simulink model "lyapanovPID"  (R2018b)
settings: Solver=VariableStepAuto  StartTime=0.0  StopTime=100  RelTol=1e-3
undefined symbols (not defined in the file or in its folder): DiscIntNeverNeededParam
libraries: simulink x1
settings Model: Creator=erfan  LastModifiedBy=erfan

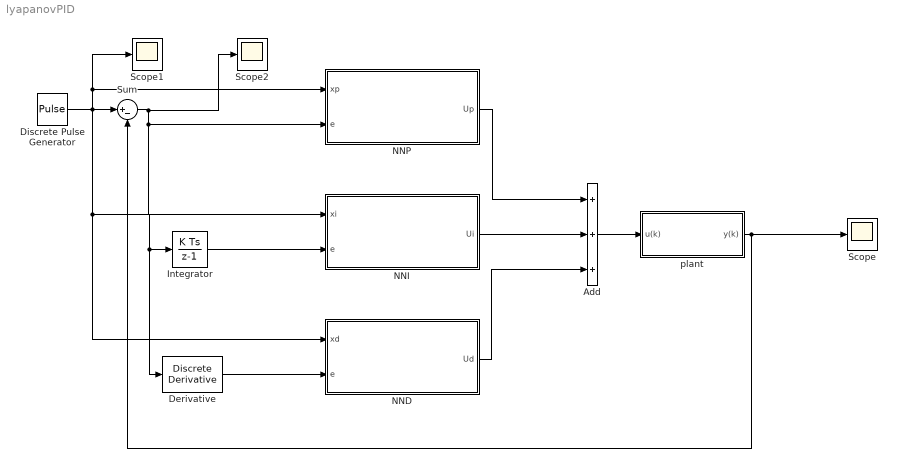
== system lyapanovPID ==
  Add : Sum  Inputs=+++
  Derivative : simulink/Quick Insert/Discrete/Discrete Derivative  gainval=1.0  ICPrevScaledInput=0.0  OutMin=[]  OutMax=[]  OutDataType=fixdt(1, 16)  OutScaling=2^-10  DoSatur=off
      settings: SourceProductName=Simulink  SourceProductBaseCode=SL
  Discrete Pulse Generator : DiscretePulseGenerator  Period=10  PulseWidth=5
  Integrator : DiscreteIntegrator  SampleTime=-1  ICPrevOutput=DiscIntNeverNeededParam  ICPrevScaledInput=DiscIntNeverNeededParam
  NND : Subsystem
  NNI : Subsystem
  NNP : Subsystem
  Scope : Scope
  Scope1 : Scope
  Scope2 : Scope
  Sum : Sum  Inputs=|+-
  plant : Subsystem
  wires:
  Derivative/1 -> NND/2(e)
  Integrator/1 -> NNI/2(e)
  NNP/1(Up) -> Add/1
  NNI/1(Ui) -> Add/2
  NND/1(Ud) -> Add/3
  Add/1 -> plant/1(u(k))
  plant/1(y(k)) -> Sum/2, Scope/1
  Sum/1 -> Scope2/1, NNP/2(e), Derivative/1, Integrator/1
  Discrete Pulse Generator/1 -> NNP/1(xp), Scope1/1, NND/1(xd), NNI/1(xi), Sum/1

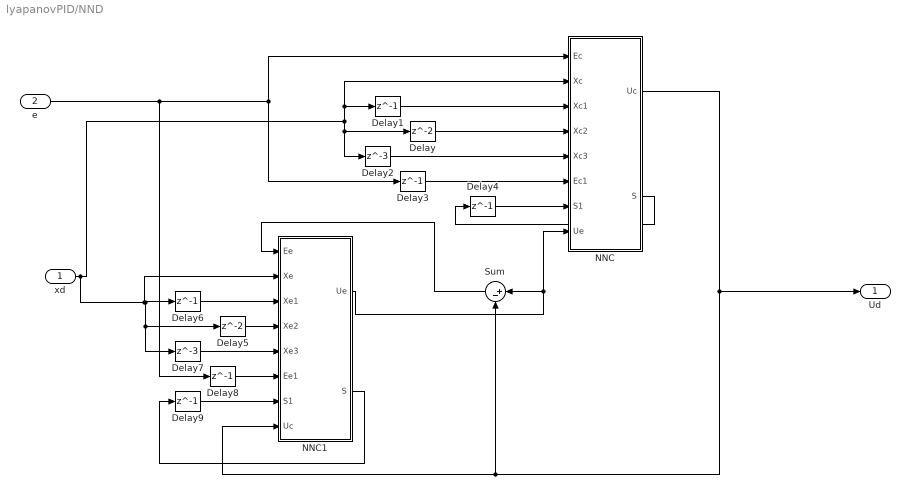
== system lyapanovPID/NND ==
  xd : Inport
  e : Inport  Port=2
  Delay : Delay
  Delay{1,3..4,6,8..9} (6 alike) : Delay  DelayLength=1
  Delay2 : Delay  DelayLength=3
  Delay5 : Delay
  Delay7 : Delay  DelayLength=3
  NNC : MATLAB Function  TreatAsAtomicUnit=on
  NNC1 : MATLAB Function  TreatAsAtomicUnit=on
  Sum : Sum  Inputs=|+-
  Ud : Outport
  wires:
  NNC1/1(Ue) -> NNC/8(Ue), Sum/1
  e/1 -> Delay8/1, Delay3/1, NNC/1(Ec)
  NNC/1(Uc) -> NNC1/8(Uc), Sum/2, Ud/1
  Sum/1 -> NNC1/1(Ee)
  Delay1/1 -> NNC/3(Xc1)
  Delay/1 -> NNC/4(Xc2)
  Delay2/1 -> NNC/5(Xc3)
  Delay3/1 -> NNC/6(Ec1)
  Delay4/1 -> NNC/7(S1)
  NNC/2(S) -> Delay4/1
  Delay7/1 -> NNC1/5(Xe3)
  xd/1 -> Delay7/1, Delay5/1, Delay6/1, NNC1/2(Xe), Delay1/1, NNC/2(Xc), Delay2/1, Delay/1
  Delay6/1 -> NNC1/3(Xe1)
  Delay8/1 -> NNC1/6(Ee1)
  Delay9/1 -> NNC1/7(S1)
  Delay5/1 -> NNC1/4(Xe2)
  NNC1/2(S) -> Delay9/1

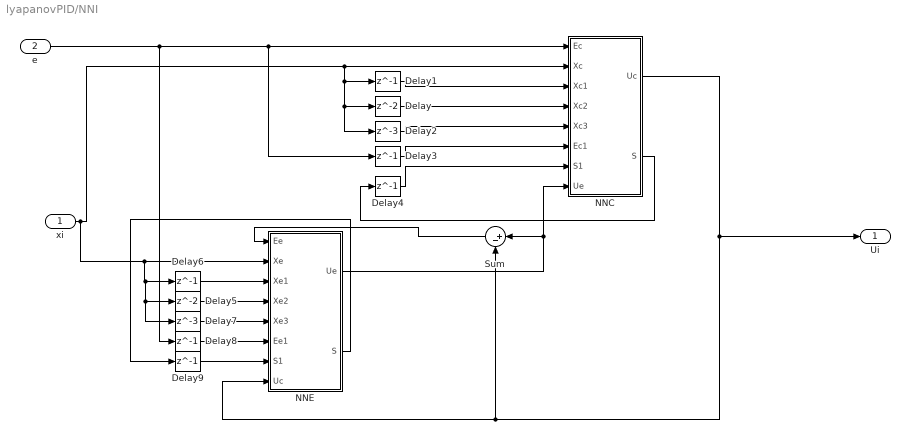
== system lyapanovPID/NNI ==
  xi : Inport
  e : Inport  Port=2
  Delay : Delay
  Delay{1,3..4,6,8..9} (6 alike) : Delay  DelayLength=1
  Delay2 : Delay  DelayLength=3
  Delay5 : Delay
  Delay7 : Delay  DelayLength=3
  NNC : MATLAB Function  TreatAsAtomicUnit=on
  NNE : MATLAB Function  TreatAsAtomicUnit=on
  Sum : Sum  Inputs=|+-
  Ui : Outport
  wires:
  NNE/1(Ue) -> Sum/1, NNC/8(Ue)
  e/1 -> Delay8/1, Delay3/1, NNC/1(Ec)
  NNC/1(Uc) -> NNE/8(Uc), Sum/2, Ui/1
  Sum/1 -> NNE/1(Ee)
  Delay1/1 -> NNC/3(Xc1)
  Delay/1 -> NNC/4(Xc2)
  Delay2/1 -> NNC/5(Xc3)
  Delay3/1 -> NNC/6(Ec1)
  Delay4/1 -> NNC/7(S1)
  NNC/2(S) -> Delay4/1
  NNE/2(S) -> Delay9/1
  Delay7/1 -> NNE/5(Xe3)
  xi/1 -> Delay7/1, Delay5/1, Delay6/1, NNE/2(Xe), Delay2/1, Delay/1, Delay1/1, NNC/2(Xc)
  Delay6/1 -> NNE/3(Xe1)
  Delay8/1 -> NNE/6(Ee1)
  Delay9/1 -> NNE/7(S1)
  Delay5/1 -> NNE/4(Xe2)

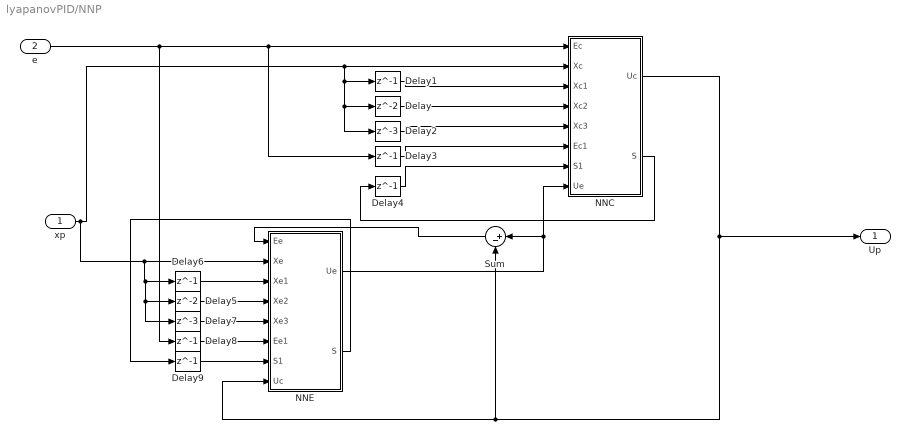
== system lyapanovPID/NNP ==
  xp : Inport
  e : Inport  Port=2
  Delay : Delay
  Delay{1,3..4,6,8..9} (6 alike) : Delay  DelayLength=1
  Delay2 : Delay  DelayLength=3
  Delay5 : Delay
  Delay7 : Delay  DelayLength=3
  NNC : MATLAB Function  TreatAsAtomicUnit=on
  NNE : MATLAB Function  TreatAsAtomicUnit=on
  Sum : Sum  Inputs=|+-
  Up : Outport
  wires:
  NNE/1(Ue) -> Sum/1, NNC/8(Ue)
  e/1 -> Delay8/1, Delay3/1, NNC/1(Ec)
  NNC/1(Uc) -> NNE/8(Uc), Sum/2, Up/1
  Sum/1 -> NNE/1(Ee)
  Delay1/1 -> NNC/3(Xc1)
  Delay/1 -> NNC/4(Xc2)
  Delay2/1 -> NNC/5(Xc3)
  Delay3/1 -> NNC/6(Ec1)
  Delay4/1 -> NNC/7(S1)
  NNC/2(S) -> Delay4/1
  NNE/2(S) -> Delay9/1
  Delay7/1 -> NNE/5(Xe3)
  xp/1 -> Delay7/1, Delay5/1, Delay6/1, NNE/2(Xe), Delay2/1, Delay/1, Delay1/1, NNC/2(Xc)
  Delay6/1 -> NNE/3(Xe1)
  Delay8/1 -> NNE/6(Ee1)
  Delay9/1 -> NNE/7(S1)
  Delay5/1 -> NNE/4(Xe2)

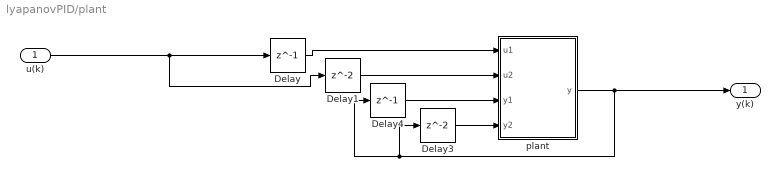
== system lyapanovPID/plant ==
  u(k) : Inport
  Delay : Delay  DelayLength=1
  Delay1 : Delay
  Delay3 : Delay
  Delay4 : Delay  DelayLength=1
  plant : MATLAB Function  TreatAsAtomicUnit=on
  y(k) : Outport
  wires:
  u(k)/1 -> Delay1/1, Delay/1
  Delay/1 -> plant/1(u1)
  Delay4/1 -> plant/3(y1)
  Delay1/1 -> plant/2(u2)
  Delay3/1 -> plant/4(y2)
  plant/1(y) -> Delay4/1, Delay3/1, y(k)/1

== matlab function lyapanovPID/NNI/NNC ==
  data: Ec input; Uc output; Xc input; Xc1 input; Xc2 input; Xc3 input; Ec1 input; S1 input; Ue input; S output
function [Uc,S] = fcn(Ec, Xc,Xc1,Xc2,Xc3,Ec1,S1, Ue)
d = Ue;
% err = Ec;
k = r;
x = Xc;
B=0.005; % this is network training rate
%% neural network initialization
N=4; % number of hidden neuron
dim=4;
Wij=0.05*rand(N,dim);  %input to hidden weights
W1j =0.05*rand(1,N);   %hidden to output weights

%% neural network 
%initializing inputs 
% x(1)=0.5;
% x(2)=0.5;
% x(3)=0.5;
% sum = 0;
%err(3) = 0;

   for j = 1:4
   % S(k,j) = tanh((Wij(1,j)*x(k-1+1) + Wij(2,j)*x(k-2+1)+Wij(3,j)*x(k-3+1)+Wij(4,j)*x(k-4+1))); % check again
   
       S(j) = tanh(Wij(j,1)*Xc+Wij(j,2)*Xc1 + Wij(j,3)*Xc2 + Wij(j,4)*Xc3);
   
   end
   
% input layer
net1 = [Xc;Xc1;Xc2;Xc3];
O1 = net1;
% hidden layyer 

net2 = Wij*O1;
O2 = [S(1),S(2),S(3),S(4)]; % not sure
%output layer
net3 = W1j.*O2;
%O3 = W1j(1,1)*S(k,1)+W1j(1,2)*S(k,2)+W1j(1,3)*S(k,3)+W1j(1,4)*S(k,4); %rewrite
%O3 = [W1j(k,1).*S(k,1);W1j(k,2).*S(k,2);W1j(k,3).*S(k,3);W1j(k,4).*S(k,4)]
u = net3(1,1)+ net3(1,2) + net3(1,3)+net3(1,4);
%err = u - x;

%% updating weights 
% Updating W1j
%d(k)=0; % must be changed
sigma = sqrt(B)*Ec1 + d;
for j = 1 :4
    W1j_new(j) = sigma  /(4*S1(j));
end
  
%Updating Wij
if i == 1
    for j = 1:4
    Wij_new(j,1) = 1/(4*Xc)*1/tanh(sigma/(4*W1j(1,j)));
    end
elseif i == 2
    for j = 1:4
    Wij_new(j,2) = 1/(4*Xc1)*1/tanh(sigma/(4*W1j(1,j)));
    end
elseif i == 3
    for j = 1:4
    Wij_new(j,3) = 1/(4*Xc2)*1/tanh(sigma/(4*W1j(1,j)));
    end
elseif i == 4
    for j = 1:4
    Wij_new(j,4) = 1/(4*Xc3)*1/tanh(sigma/(4*W1j(1,j)));
    end
end
% for i = 1:4
%     for j = 1:4
%         Wij_new(j,i) = 1/(4*x(k-i+1))*1/tanh(sigma/(4*W1j(1,j))); % Not OK
%     end
% 
% end
Wij = Wij_new;
W1j = W1j_new;



Uc = u;

== matlab function lyapanovPID/NNP/NNC ==
  data: Ec input; Uc output; Xc input; Xc1 input; Xc2 input; Xc3 input; Ec1 input; S1 input; Ue input; S output
function [Uc,S] = fcn(Ec, Xc,Xc1,Xc2,Xc3,Ec1,S1, Ue)
d = Ue;
% err = Ec;
k = r;
x = Xc;
B=0.005; % this is network training rate
%% neural network initialization
N=4; % number of hidden neuron
dim=4;
Wij=0.05*rand(N,dim);  %input to hidden weights
W1j =0.05*rand(1,N);   %hidden to output weights

%% neural network 
%initializing inputs 
% x(1)=0.5;
% x(2)=0.5;
% x(3)=0.5;
% sum = 0;
%err(3) = 0;

   for j = 1:4
   % S(k,j) = tanh((Wij(1,j)*x(k-1+1) + Wij(2,j)*x(k-2+1)+Wij(3,j)*x(k-3+1)+Wij(4,j)*x(k-4+1))); % check again
   
       S(j) = tanh(Wij(j,1)*Xc+Wij(j,2)*Xc1 + Wij(j,3)*Xc2 + Wij(j,4)*Xc3);
   
   end
   
% input layer
net1 = [Xc;Xc1;Xc2;Xc3];
O1 = net1;
% hidden layyer 

net2 = Wij*O1;
O2 = [S(1),S(2),S(3),S(4)]; % not sure
%output layer
net3 = W1j.*O2;
%O3 = W1j(1,1)*S(k,1)+W1j(1,2)*S(k,2)+W1j(1,3)*S(k,3)+W1j(1,4)*S(k,4); %rewrite
%O3 = [W1j(k,1).*S(k,1);W1j(k,2).*S(k,2);W1j(k,3).*S(k,3);W1j(k,4).*S(k,4)]
u = net3(1,1)+ net3(1,2) + net3(1,3)+net3(1,4);
%err = u - x;

%% updating weights 
% Updating W1j
%d(k)=0; % must be changed
sigma = sqrt(B)*Ec1 + d;
for j = 1 :4
    W1j_new(j) = sigma  /(4*S1(j));
end
  
%Updating Wij
if i == 1
    for j = 1:4
    Wij_new(j,1) = 1/(4*Xc)*1/tanh(sigma/(4*W1j(1,j)));
    end
elseif i == 2
    for j = 1:4
    Wij_new(j,2) = 1/(4*Xc1)*1/tanh(sigma/(4*W1j(1,j)));
    end
elseif i == 3
    for j = 1:4
    Wij_new(j,3) = 1/(4*Xc2)*1/tanh(sigma/(4*W1j(1,j)));
    end
elseif i == 4
    for j = 1:4
    Wij_new(j,4) = 1/(4*Xc3)*1/tanh(sigma/(4*W1j(1,j)));
    end
end
% for i = 1:4
%     for j = 1:4
%         Wij_new(j,i) = 1/(4*x(k-i+1))*1/tanh(sigma/(4*W1j(1,j))); % Not OK
%     end
% 
% end
Wij = Wij_new;
W1j = W1j_new;



Uc = u;

== matlab function lyapanovPID/plant/plant ==
  data: u1 input; y output; u2 input; y1 input; y2 input
function y = fcn(u1,u2,y1,y2)

y = (0.8*y1 + 2*u1)/(1 + 1.5*y2*u2)

== matlab function lyapanovPID/NNP/NNE ==
  data: Ee input; Ue output; Xe input; Xe1 input; Xe2 input; Xe3 input; Ee1 input; S1 input; Uc input; S output
function [Ue,S] = fcn(Ee, Xe,Xe1,Xe2,Xe3,Ee1,S1, Uc)
d = Uc;
% err = Ec;
k = r;
x = Xe;
B=0.005; % this is network training rate
%% neural network initialization
N=4; % number of hidden neuron
dim=4;
Wij=0.05*rand(N,dim);  %input to hidden weights
W1j =0.05*rand(1,N);   %hidden to output weights

%% neural network 
%initializing inputs 
% x(1)=0.5;
% x(2)=0.5;
% x(3)=0.5;
% sum = 0;
%err(3) = 0;

   for j = 1:4
   % S(k,j) = tanh((Wij(1,j)*x(k-1+1) + Wij(2,j)*x(k-2+1)+Wij(3,j)*x(k-3+1)+Wij(4,j)*x(k-4+1))); % check again
   
       S(j) = tanh(Wij(j,1)*Xe+Wij(j,2)*Xe1 + Wij(j,3)*Xe2 + Wij(j,4)*Xe3);
   
   end
   
% input layer
net1 = [Xe;Xe1;Xe2;Xe3];
O1 = net1;
% hidden layyer 

net2 = Wij*O1;
O2 = [S(1),S(2),S(3),S(4)]; % not sure
%output layer
net3 = W1j.*O2;
%O3 = W1j(1,1)*S(k,1)+W1j(1,2)*S(k,2)+W1j(1,3)*S(k,3)+W1j(1,4)*S(k,4); %rewrite
%O3 = [W1j(k,1).*S(k,1);W1j(k,2).*S(k,2);W1j(k,3).*S(k,3);W1j(k,4).*S(k,4)]
u = net3(1,1)+ net3(1,2) + net3(1,3)+net3(1,4);
%err = u - x;

%% updating weights 
% Updating W1j
%d(k)=0; % must be changed
sigma = sqrt(B)*Ee1 + d;
for j = 1 :4
    W1j_new(j) = sigma  /(4*S1(j));
end
  
%Updating Wij
if i == 1
    for j = 1:4
    Wij_new(j,1) = 1/(4*Xe)*1/tanh(sigma/(4*W1j(1,j)));
    end
elseif i == 2
    for j = 1:4
    Wij_new(j,2) = 1/(4*Xe1)*1/tanh(sigma/(4*W1j(1,j)));
    end
elseif i == 3
    for j = 1:4
    Wij_new(j,3) = 1/(4*Xe2)*1/tanh(sigma/(4*W1j(1,j)));
    end
elseif i == 4
    for j = 1:4
    Wij_new(j,4) = 1/(4*Xe3)*1/tanh(sigma/(4*W1j(1,j)));
    end
end
% for i = 1:4
%     for j = 1:4
%         Wij_new(j,i) = 1/(4*x(k-i+1))*1/tanh(sigma/(4*W1j(1,j))); % Not OK
%     end
% 
% end
Wij = Wij_new;
W1j = W1j_new;



Ue = u;

== matlab function lyapanovPID/NNI/NNE ==
  data: Ee input; Ue output; Xe input; Xe1 input; Xe2 input; Xe3 input; Ee1 input; S1 input; Uc input; S output
function [Ue,S] = fcn(Ee, Xe,Xe1,Xe2,Xe3,Ee1,S1, Uc)
d = Uc;
% err = Ec;
k = r;
x = Xe;
B=0.005; % this is network training rate
%% neural network initialization
N=4; % number of hidden neuron
dim=4;
Wij=0.05*rand(N,dim);  %input to hidden weights
W1j =0.05*rand(1,N);   %hidden to output weights

%% neural network 
%initializing inputs 
% x(1)=0.5;
% x(2)=0.5;
% x(3)=0.5;
% sum = 0;
%err(3) = 0;

   for j = 1:4
   % S(k,j) = tanh((Wij(1,j)*x(k-1+1) + Wij(2,j)*x(k-2+1)+Wij(3,j)*x(k-3+1)+Wij(4,j)*x(k-4+1))); % check again
   
       S(j) = tanh(Wij(j,1)*Xe+Wij(j,2)*Xe1 + Wij(j,3)*Xe2 + Wij(j,4)*Xe3);
   
   end
   
% input layer
net1 = [Xe;Xe1;Xe2;Xe3];
O1 = net1;
% hidden layyer 

net2 = Wij*O1;
O2 = [S(1),S(2),S(3),S(4)]; % not sure
%output layer
net3 = W1j.*O2;
%O3 = W1j(1,1)*S(k,1)+W1j(1,2)*S(k,2)+W1j(1,3)*S(k,3)+W1j(1,4)*S(k,4); %rewrite
%O3 = [W1j(k,1).*S(k,1);W1j(k,2).*S(k,2);W1j(k,3).*S(k,3);W1j(k,4).*S(k,4)]
u = net3(1,1)+ net3(1,2) + net3(1,3)+net3(1,4);
%err = u - x;

%% updating weights 
% Updating W1j
%d(k)=0; % must be changed
sigma = sqrt(B)*Ee1 + d;
for j = 1 :4
    W1j_new(j) = sigma  /(4*S1(j));
end
  
%Updating Wij
if i == 1
    for j = 1:4
    Wij_new(j,1) = 1/(4*Xe)*1/tanh(sigma/(4*W1j(1,j)));
    end
elseif i == 2
    for j = 1:4
    Wij_new(j,2) = 1/(4*Xe1)*1/tanh(sigma/(4*W1j(1,j)));
    end
elseif i == 3
    for j = 1:4
    Wij_new(j,3) = 1/(4*Xe2)*1/tanh(sigma/(4*W1j(1,j)));
    end
elseif i == 4
    for j = 1:4
    Wij_new(j,4) = 1/(4*Xe3)*1/tanh(sigma/(4*W1j(1,j)));
    end
end
% for i = 1:4
%     for j = 1:4
%         Wij_new(j,i) = 1/(4*x(k-i+1))*1/tanh(sigma/(4*W1j(1,j))); % Not OK
%     end
% 
% end
Wij = Wij_new;
W1j = W1j_new;



Ue = u;

== matlab function lyapanovPID/NND/NNC ==
  data: Ec input; Uc output; Xc input; Xc1 input; Xc2 input; Xc3 input; Ec1 input; S1 input; Ue input; S output
function [Uc,S] = fcn(Ec, Xc,Xc1,Xc2,Xc3,Ec1,S1, Ue)
d = Ue;
% err = Ec;
k = r;
x = Xc;
B=0.005; % this is network training rate
%% neural network initialization
N=4; % number of hidden neuron
dim=4;
Wij=0.05*rand(N,dim);  %input to hidden weights
W1j =0.05*rand(1,N);   %hidden to output weights

%% neural network 
%initializing inputs 
% x(1)=0.5;
% x(2)=0.5;
% x(3)=0.5;
% sum = 0;
%err(3) = 0;

   for j = 1:4
   % S(k,j) = tanh((Wij(1,j)*x(k-1+1) + Wij(2,j)*x(k-2+1)+Wij(3,j)*x(k-3+1)+Wij(4,j)*x(k-4+1))); % check again
   
       S(j) = tanh(Wij(j,1)*Xc+Wij(j,2)*Xc1 + Wij(j,3)*Xc2 + Wij(j,4)*Xc3);
   
   end
   
% input layer
net1 = [Xc;Xc1;Xc2;Xc3];
O1 = net1;
% hidden layyer 

net2 = Wij*O1;
O2 = [S(1),S(2),S(3),S(4)]; % not sure
%output layer
net3 = W1j.*O2;
%O3 = W1j(1,1)*S(k,1)+W1j(1,2)*S(k,2)+W1j(1,3)*S(k,3)+W1j(1,4)*S(k,4); %rewrite
%O3 = [W1j(k,1).*S(k,1);W1j(k,2).*S(k,2);W1j(k,3).*S(k,3);W1j(k,4).*S(k,4)]
u = net3(1,1)+ net3(1,2) + net3(1,3)+net3(1,4);
%err = u - x;

%% updating weights 
% Updating W1j
%d(k)=0; % must be changed
sigma = sqrt(B)*Ec1 + d;
for j = 1 :4
    W1j_new(j) = sigma  /(4*S1(j));
end
  
%Updating Wij
if i == 1
    for j = 1:4
    Wij_new(j,1) = 1/(4*Xc)*1/tanh(sigma/(4*W1j(1,j)));
    end
elseif i == 2
    for j = 1:4
    Wij_new(j,2) = 1/(4*Xc1)*1/tanh(sigma/(4*W1j(1,j)));
    end
elseif i == 3
    for j = 1:4
    Wij_new(j,3) = 1/(4*Xc2)*1/tanh(sigma/(4*W1j(1,j)));
    end
elseif i == 4
    for j = 1:4
    Wij_new(j,4) = 1/(4*Xc3)*1/tanh(sigma/(4*W1j(1,j)));
    end
end
% for i = 1:4
%     for j = 1:4
%         Wij_new(j,i) = 1/(4*x(k-i+1))*1/tanh(sigma/(4*W1j(1,j))); % Not OK
%     end
% 
% end
Wij = Wij_new;
W1j = W1j_new;



Uc = u;

== matlab function lyapanovPID/NND/NNC1 ==
  data: Ee input; Ue output; Xe input; Xe1 input; Xe2 input; Xe3 input; Ee1 input; S1 input; Uc input; S output
function [Ue,S] = fcn(Ee, Xe,Xe1,Xe2,Xe3,Ee1,S1, Uc)
d = Uc;
% err = Ec;
k = r;
x = Xe;
B=0.005; % this is network training rate
%% neural network initialization
N=4; % number of hidden neuron
dim=4;
Wij=0.05*rand(N,dim);  %input to hidden weights
W1j =0.05*rand(1,N);   %hidden to output weights

%% neural network 
%initializing inputs 
% x(1)=0.5;
% x(2)=0.5;
% x(3)=0.5;
% sum = 0;
%err(3) = 0;

   for j = 1:4
   % S(k,j) = tanh((Wij(1,j)*x(k-1+1) + Wij(2,j)*x(k-2+1)+Wij(3,j)*x(k-3+1)+Wij(4,j)*x(k-4+1))); % check again
   
       S(j) = tanh(Wij(j,1)*Xe+Wij(j,2)*Xe1 + Wij(j,3)*Xe2 + Wij(j,4)*Xe3);
   
   end
   
% input layer
net1 = [Xe;Xe1;Xe2;Xe3];
O1 = net1;
% hidden layyer 

net2 = Wij*O1;
O2 = [S(1),S(2),S(3),S(4)]; % not sure
%output layer
net3 = W1j.*O2;
%O3 = W1j(1,1)*S(k,1)+W1j(1,2)*S(k,2)+W1j(1,3)*S(k,3)+W1j(1,4)*S(k,4); %rewrite
%O3 = [W1j(k,1).*S(k,1);W1j(k,2).*S(k,2);W1j(k,3).*S(k,3);W1j(k,4).*S(k,4)]
u = net3(1,1)+ net3(1,2) + net3(1,3)+net3(1,4);
%err = u - x;

%% updating weights 
% Updating W1j
%d(k)=0; % must be changed
sigma = sqrt(B)*Ee1 + d;
for j = 1 :4
    W1j_new(j) = sigma  /(4*S1(j));
end
  
%Updating Wij
if i == 1
    for j = 1:4
    Wij_new(j,1) = 1/(4*Xe)*1/tanh(sigma/(4*W1j(1,j)));
    end
elseif i == 2
    for j = 1:4
    Wij_new(j,2) = 1/(4*Xe1)*1/tanh(sigma/(4*W1j(1,j)));
    end
elseif i == 3
    for j = 1:4
    Wij_new(j,3) = 1/(4*Xe2)*1/tanh(sigma/(4*W1j(1,j)));
    end
elseif i == 4
    for j = 1:4
    Wij_new(j,4) = 1/(4*Xe3)*1/tanh(sigma/(4*W1j(1,j)));
    end
end
% for i = 1:4
%     for j = 1:4
%         Wij_new(j,i) = 1/(4*x(k-i+1))*1/tanh(sigma/(4*W1j(1,j))); % Not OK
%     end
% 
% end
Wij = Wij_new;
W1j = W1j_new;



Ue = u;
